simulink model "prob7"  (R2020b)
settings: Solver=VariableStepAuto  StartTime=0.0  StopTime=10.0  RelTol=1e-3
undefined symbols (not defined in the file): a0, a1, a2, b0, b1, b2
settings Model: Creator=AVM  LastModifiedBy=AVM

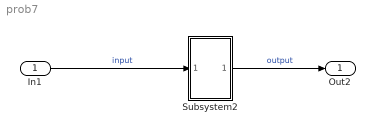
== system prob7 ==
  In1 : Inport
  Subsystem2 : Subsystem
  Out2 : Outport
  wires:
  In1/1 -> Subsystem2/1(In1)  "input"
  Subsystem2/1(Out1) -> Out2/1  "output"

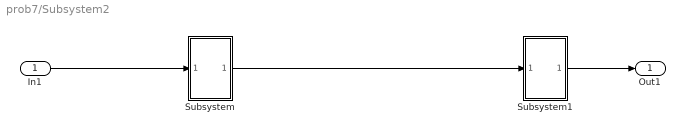
== system prob7/Subsystem2 ==
  In1 : Inport
  Subsystem : Subsystem
  Subsystem1 : Subsystem
  Out1 : Outport
  wires:
  Subsystem/1(Out1) -> Subsystem1/1(In1)
  Subsystem1/1(Out1) -> Out1/1
  In1/1 -> Subsystem/1(In1)

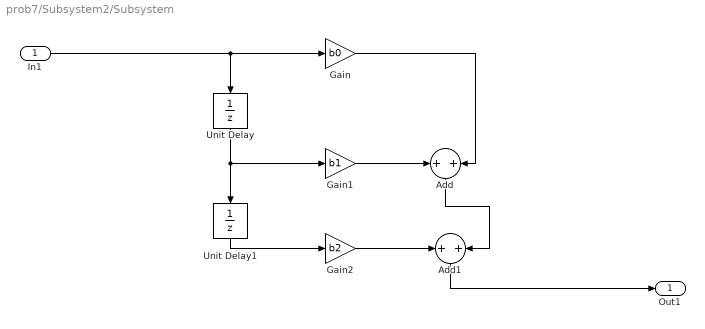
== system prob7/Subsystem2/Subsystem ==
  In1 : Inport
  Add : Sum
  Add1 : Sum
  Gain : Gain  Gain=b0
  Gain1 : Gain  Gain=b1
  Gain2 : Gain  Gain=b2
  Unit Delay : UnitDelay  SampleTime=-1  HasFrameUpgradeWarning=on
  Unit Delay1 : UnitDelay  SampleTime=-1  HasFrameUpgradeWarning=on
  Out1 : Outport
  wires:
  In1/1 -> Gain/1, Unit Delay/1
  Gain/1 -> Add/2
  Unit Delay/1 -> Gain1/1, Unit Delay1/1
  Unit Delay1/1 -> Gain2/1
  Gain2/1 -> Add1/1
  Gain1/1 -> Add/1
  Add/1 -> Add1/2
  Add1/1 -> Out1/1

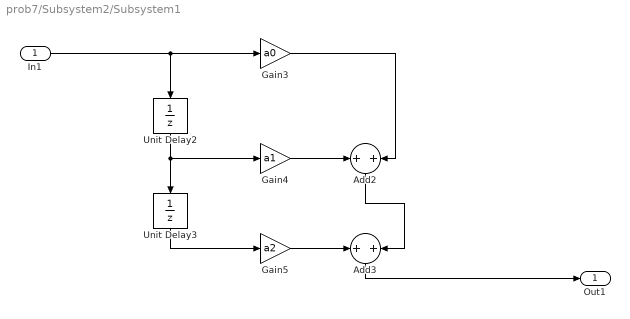
== system prob7/Subsystem2/Subsystem1 ==
  In1 : Inport
  Add2 : Sum
  Add3 : Sum
  Gain3 : Gain  Gain=a0
  Gain4 : Gain  Gain=a1
  Gain5 : Gain  Gain=a2
  Unit Delay2 : UnitDelay  SampleTime=-1  HasFrameUpgradeWarning=on
  Unit Delay3 : UnitDelay  SampleTime=-1  HasFrameUpgradeWarning=on
  Out1 : Outport
  wires:
  Gain3/1 -> Add2/2
  In1/1 -> Gain3/1, Unit Delay2/1
  Unit Delay3/1 -> Gain5/1
  Unit Delay2/1 -> Unit Delay3/1, Gain4/1
  Gain4/1 -> Add2/1
  Add2/1 -> Add3/2
  Gain5/1 -> Add3/1
  Add3/1 -> Out1/1
